simulink model "robot"  (Simulink 9.0)
settings: Solver=FixedStepDiscrete  StartTime=0.0  StopTime=inf  FixedStep=0.022  RelTol=1e-3  EnableMultiTasking=on
values from neighbouring files (symbols this model uses):
  s = zc-d1    [ArticuledManipulator_Ik.m]
undefined symbols (not defined in the file or in its folder): RV
libraries: mblibv1 x37, vrlib x8, simulink x1
settings Model: Creator=Mircea  LastModifiedBy=Rodrigo Chi
settings DataIOCC: LimitDataPoints=on  SignalLoggingSaveFormat=ModelDataLogs
settings OptimizationCC: ExpressionDepthLimit=2147483647
settings DebuggingCC: SolverPrmCheckMsg=warning  FcnCallInpInsideContextMsg=warning  StateNameClashWarn=warning
settings SFSimCC: SimParseCustomCode=off
settings GRTTargetCC: GeneratePreprocessorConditionals=Disable all  CombineOutputUpdateFcns=off  GRTInterface=on
settings ConfigComp: CovSFcnEnable=off
settings SimscapeCC: SimscapeNormalizeSystem=off
settings ConfigurationSet: Description=SimMechanics 2G

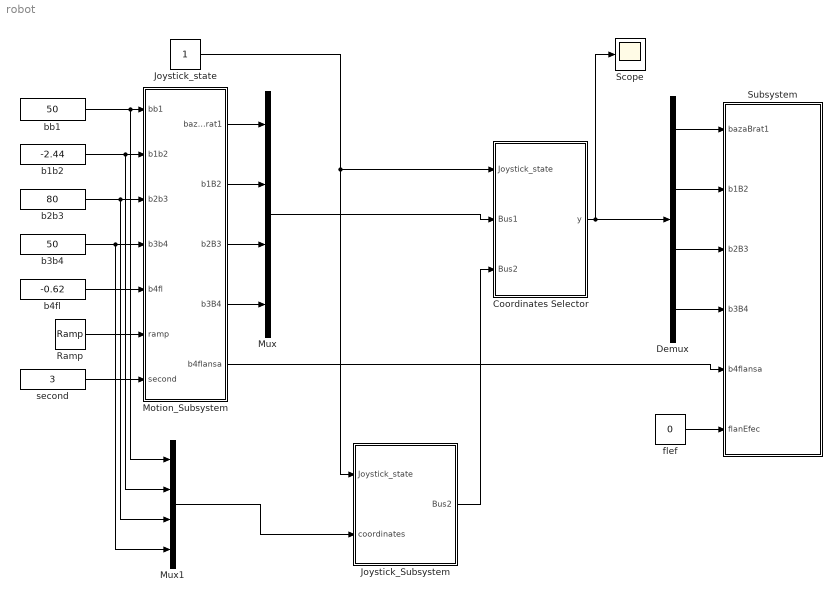
== system robot ==
  "Coordinates Selector " : MATLAB Function  TreatAsAtomicUnit=on
  Demux : Demux
  Joystick_Subsystem : Subsystem
  Joystick_state : Constant
  Motion_Subsystem : Subsystem
  Mux : Mux
  Mux1 : Mux
  Ramp : simulink/Sources/Ramp  slope=25  start=0  X0=0
  Scope : Scope
  Subsystem : Subsystem
  b1b2 : Constant  Value=-2.44
  b2b3 : Constant  Value=80
  b3b4 : Constant  Value=50
  b4fl : Constant  Value=-0.62
  bb1 : Constant  Value=50
  flef : Constant  Value=0
  second : Constant  Value=3
  wires:
  b1b2/1 -> Motion_Subsystem/2(b1b2), Mux1/2
  b2b3/1 -> Motion_Subsystem/3(b2b3), Mux1/3
  b3b4/1 -> Motion_Subsystem/4(b3b4), Mux1/4
  b4fl/1 -> Motion_Subsystem/5(b4fl)
  Ramp/1 -> Motion_Subsystem/6(ramp)
  bb1/1 -> Motion_Subsystem/1(bb1), Mux1/1
  flef/1 -> Subsystem/6(flanEfec)
  second/1 -> Motion_Subsystem/7(second)
  Motion_Subsystem/5(b4flansa) -> Subsystem/5(b4flansa)
  Motion_Subsystem/1(bazaBrat1) -> Mux/1
  Motion_Subsystem/2(b1B2) -> Mux/2
  Motion_Subsystem/3(b2B3) -> Mux/3
  Motion_Subsystem/4(b3B4) -> Mux/4
  Mux/1 -> "Coordinates Selector "/2(Bus1)
  Joystick_state/1 -> "Coordinates Selector "/1(Joystick_state), Joystick_Subsystem/1(Joystick_state)
  "Coordinates Selector "/1(y) -> Demux/1, Scope/1
  Demux/1 -> Subsystem/1(bazaBrat1)
  Demux/2 -> Subsystem/2(b1B2)
  Demux/3 -> Subsystem/3(b2B3)
  Demux/4 -> Subsystem/4(b3B4)
  Mux1/1 -> Joystick_Subsystem/2(coordinates)
  Joystick_Subsystem/1(Bus2) -> "Coordinates Selector "/3(Bus2)

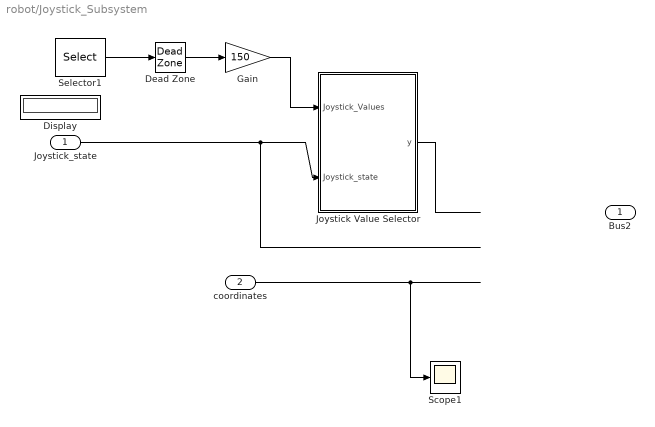
== system robot/Joystick_Subsystem ==
  Joystick_state : Inport
  coordinates : Inport  Port=2
  Dead Zone : DeadZone  SaturateOnIntegerOverflow=on
  Display : Display
  Gain : Gain  Gain=150
  "Joystick Value Selector " : MATLAB Function  TreatAsAtomicUnit=on
  Scope1 : Scope
  Selector1 : Selector  InputPortWidth=8  IndexOptions=Index vector (dialog)  Indices=[1 2 3 4]  OutputSizes=1
  Bus2 : Outport
  wires:
  ? -> Selector1/1
  Selector1/1 -> Dead Zone/1
  Dead Zone/1 -> Gain/1
  coordinates/1 -> Scope1/1
  Joystick_state/1 -> "Joystick Value Selector "/2(Joystick_state)
  Gain/1 -> "Joystick Value Selector "/1(Joystick_Values)
  "Joystick Value Selector "/1(y) -> ?
  ? -> Bus2/1
  ? -> Display/1

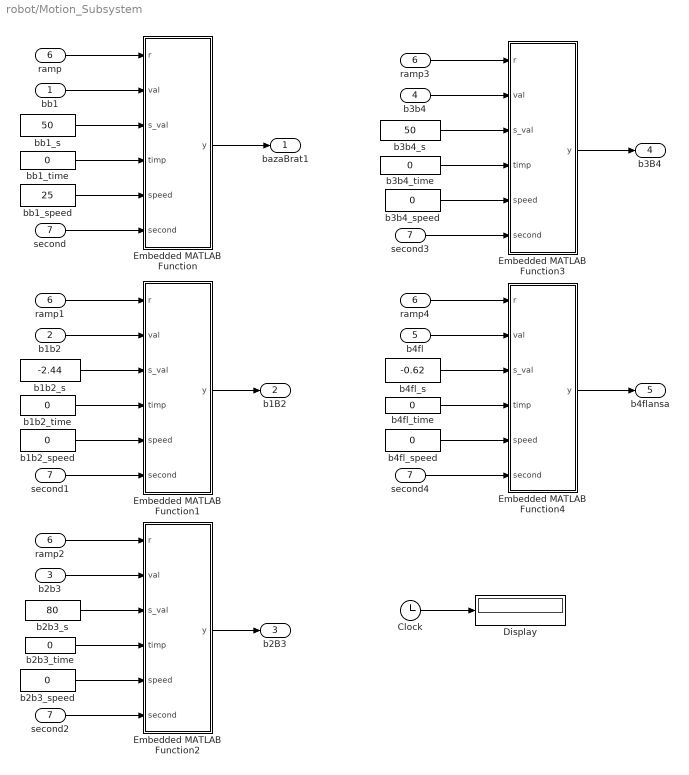
== system robot/Motion_Subsystem ==
  bb1 : Inport
  b1b2 : Inport  Port=2
  b2b3 : Inport  Port=3
  b3b4 : Inport  Port=4
  b4fl : Inport  Port=5
  ramp : Inport  Port=6
  second : Inport  Port=7
  Clock : Clock
  Display : Display
  Embedded MATLAB Function : MATLAB Function  TreatAsAtomicUnit=on
  Embedded MATLAB Function1 : MATLAB Function  TreatAsAtomicUnit=on
  Embedded MATLAB Function2 : MATLAB Function  TreatAsAtomicUnit=on
  Embedded MATLAB Function3 : MATLAB Function  TreatAsAtomicUnit=on
  Embedded MATLAB Function4 : MATLAB Function  TreatAsAtomicUnit=on
  b1b2_s : Constant  Value=-2.44
  b1b2_speed : Constant  Value=0
  b1b2_time : Constant  Value=0
  b2b3_s : Constant  Value=80
  b2b3_speed : Constant  Value=0
  b2b3_time : Constant  Value=0
  b3b4_s : Constant  Value=50
  b3b4_speed : Constant  Value=0
  b3b4_time : Constant  Value=0
  b4fl_s : Constant  Value=-0.62
  b4fl_speed : Constant  Value=0
  b4fl_time : Constant  Value=0
  bb1_s : Constant  Value=50
  bb1_speed : Constant  Value=25
  bb1_time : Constant  Value=0
  ramp{1..4} (4 alike) : InportShadow  Port=6
  second{1..4} (4 alike) : InportShadow  Port=7
  bazaBrat1 : Outport
  b1B2 : Outport  Port=2
  b2B3 : Outport  Port=3
  b3B4 : Outport  Port=4
  b4flansa : Outport  Port=5
  wires:
  ramp/1 -> Embedded MATLAB Function/1(r)
  Clock/1 -> Display/1
  b4fl_time/1 -> Embedded MATLAB Function4/4(timp)
  b4fl_s/1 -> Embedded MATLAB Function4/3(s_val)
  ramp4/1 -> Embedded MATLAB Function4/1(r)
  Embedded MATLAB Function4/1(y) -> b4flansa/1
  b4fl/1 -> Embedded MATLAB Function4/2(val)
  ramp3/1 -> Embedded MATLAB Function3/1(r)
  b3b4_time/1 -> Embedded MATLAB Function3/4(timp)
  b3b4_s/1 -> Embedded MATLAB Function3/3(s_val)
  Embedded MATLAB Function3/1(y) -> b3B4/1
  b3b4/1 -> Embedded MATLAB Function3/2(val)
  b2b3_time/1 -> Embedded MATLAB Function2/4(timp)
  b2b3_s/1 -> Embedded MATLAB Function2/3(s_val)
  ramp2/1 -> Embedded MATLAB Function2/1(r)
  Embedded MATLAB Function2/1(y) -> b2B3/1
  b2b3/1 -> Embedded MATLAB Function2/2(val)
  b1b2_time/1 -> Embedded MATLAB Function1/4(timp)
  b1b2_s/1 -> Embedded MATLAB Function1/3(s_val)
  ramp1/1 -> Embedded MATLAB Function1/1(r)
  Embedded MATLAB Function1/1(y) -> b1B2/1
  b1b2/1 -> Embedded MATLAB Function1/2(val)
  bb1_time/1 -> Embedded MATLAB Function/4(timp)
  bb1_s/1 -> Embedded MATLAB Function/3(s_val)
  Embedded MATLAB Function/1(y) -> bazaBrat1/1
  bb1/1 -> Embedded MATLAB Function/2(val)
  bb1_speed/1 -> Embedded MATLAB Function/5(speed)
  b3b4_speed/1 -> Embedded MATLAB Function3/5(speed)
  b4fl_speed/1 -> Embedded MATLAB Function4/5(speed)
  b2b3_speed/1 -> Embedded MATLAB Function2/5(speed)
  b1b2_speed/1 -> Embedded MATLAB Function1/5(speed)
  second/1 -> Embedded MATLAB Function/6(second)
  second4/1 -> Embedded MATLAB Function4/6(second)
  second3/1 -> Embedded MATLAB Function3/6(second)
  second2/1 -> Embedded MATLAB Function2/6(second)
  second1/1 -> Embedded MATLAB Function1/6(second)

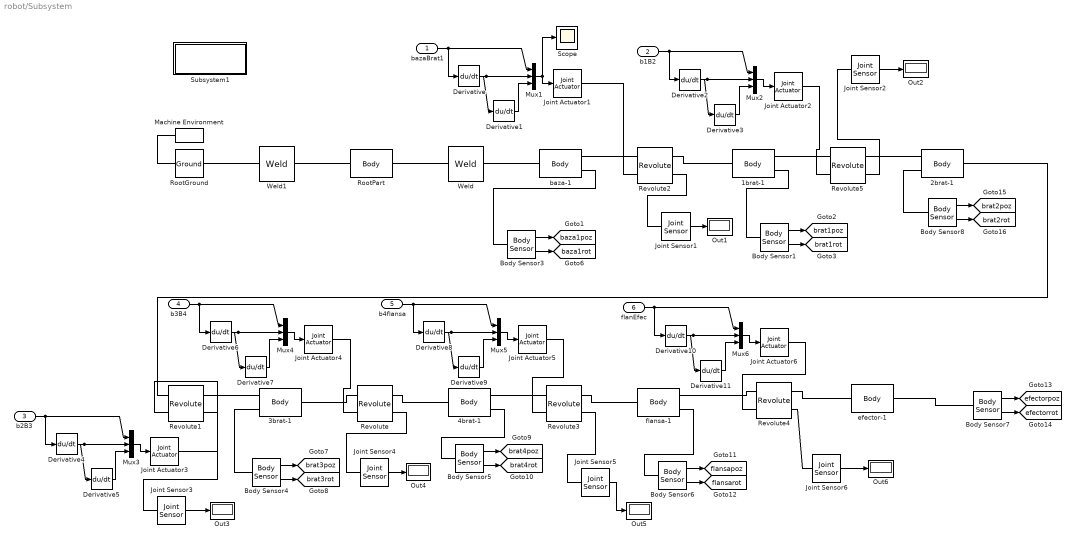
== system robot/Subsystem ==
  bazaBrat1 : Inport
  b1B2 : Inport  Port=2
  b2B3 : Inport  Port=3
  b3B4 : Inport  Port=4
  b4flansa : Inport  Port=5
  flanEfec : Inport  Port=6
  1brat-1 : mblibv1/Bodies/Body  LConnTagsString=CS2  RConnTagsString=CS3|CS4  UpdateFromCAD=on  DialogClass=MechanicalBodyBlock  Mass=2.25015  MassUnits=kg  InertiaUnits=kg*m^2  Inertia=[0.00885227,-5.51348e-008,-0.000219712;-5.51348e-008,0.00930047,6.21532e-009;-0.000219712,6.21532e-009,0.00500541]  Shape=Cylinder  ShapeDims=[1 1]  ShapeUnits=m  ShapeUse=false  Density=1  DensityUnits=kg/m^3  DensityUse=false  GraphicsMode=GFXFILE  GraphicsFileName=robot_nou - 1brat-1.STL  BodyColorSelMode=COLORPALETTE  BodyColor=[0.75294 0.75294 0.75294]  AttachedToCS=CS1  CG=Right$CG$[0.00726331 0.0794388 -8.78869e-008]$WORLD$WORLD$m$[-1 0 0;0 0 1;0 1 0]$3x3 Transform$rad$WORLD$false$none  WorkingFrames=Right$CS1$[0 -0.00299998 0]$WORLD$WORLD$m$[-1 0 0;0 0 1;0 1 0]$3x3 Transform$rad$WORLD$false$none#Left$CS2$[-1.38778e-017 2.5e-008 5.8564e-016]$WORLD$WORLD$m$[1 0 0;0 1 0;0 0 1]$3x3 Transform$rad$WORLD$true$none#Right$CS3$[0 0.1295 -0.0448145]$WORLD$WORLD$m$[1 0 0;0 1 0;0 0 1]$3x3 Transform$rad$WORLD$true$none#Right$CS4$[0 0 0]$WORLD$WORLD$m$[1 0 0;0 1 0;0 0 1]$3x3 Transform$rad$WORLD$true$none  CGPos=[0.00726331 0.0794388 -8.78869e-008]  CGRot=[-1 0 0;0 0 1;0 1 0]  CS0Pos=[]  CS0Rot=[]  CS1Pos=[0 -0.00299998 0]  CS1Rot=[-1 0 0;0 0 1;0 1 0]  CS2Pos=[-1.38778e-017 2.5e-008 5.8564e-016]  CS2Rot=[1 0 0;0 1 0;0 0 1]  CS3Pos=[0 0.1295 -0.0448145]  CS3Rot=[1 0 0;0 1 0;0 0 1]  CS4Pos=[0 0 0]  CS4Rot=[1 0 0;0 1 0;0 0 1]  CS5Pos=[]  CS5Rot=[]  CS6Pos=[]  CS6Rot=[]  CS7Pos=[]  CS7Rot=[]  CS8Pos=[]  CS8Rot=[]  CS9Pos=[]  CS9Rot=[]  CS10Pos=[]  CS10Rot=[]  CS11Pos=[]  CS11Rot=[]  CS12Pos=[]  CS12Rot=[]  CS13Pos=[]  CS13Rot=[]  CS14Pos=[]  CS14Rot=[]  CS15Pos=[]  CS15Rot=[]  CS16Pos=[]  CS16Rot=[]  CS17Pos=[]  CS17Rot=[]  CS18Pos=[]  CS18Rot=[]  CS19Pos=[]  CS19Rot=[]  CS20Pos=[]  CS20Rot=[]
      settings: SourceProductName=Simscape Multibody  SourceProductBaseCode=MS
  2brat-1 : mblibv1/Bodies/Body  LConnTagsString=CS3|CS4  RConnTagsString=CS2  UpdateFromCAD=on  DialogClass=MechanicalBodyBlock  Mass=3.62743  MassUnits=kg  InertiaUnits=kg*m^2  Inertia=[0.0393757,-7.68618e-009,0.000126615;-7.68618e-009,0.0293486,-4.48119e-008;0.000126615,-4.48119e-008,0.0153003]  Shape=Cylinder  ShapeDims=[1 1]  ShapeUnits=m  ShapeUse=false  Density=1  DensityUnits=kg/m^3  DensityUse=false  GraphicsMode=GFXFILE  GraphicsFileName=robot_nou - 2brat-1.STL  BodyColorSelMode=COLORPALETTE  BodyColor=[0.75294 0.75294 0.75294]  AttachedToCS=CS1  CG=Right$CG$[-0.000659844 0.24353 1.10558e-006]$WORLD$WORLD$m$[1 0 0;0 0 1;0 -1 0]$3x3 Transform$rad$WORLD$false$none  WorkingFrames=Right$CS1$[0 0.1295 0]$WORLD$WORLD$m$[1 0 0;0 0 1;0 -1 0]$3x3 Transform$rad$WORLD$false$none#Right$CS2$[0 0.3795 0.0880007]$WORLD$WORLD$m$[1 0 0;0 1 0;0 0 1]$3x3 Transform$rad$WORLD$true$none#Left$CS3$[0 0.1295 -0.0448145]$WORLD$WORLD$m$[1 0 0;0 1 0;0 0 1]$3x3 Transform$rad$WORLD$true$none#Left$CS4$[0 0 0]$WORLD$WORLD$m$[1 0 0;0 1 0;0 0 1]$3x3 Transform$rad$WORLD$true$none  CGPos=[-0.000659844 0.24353 1.10558e-006]  CGRot=[1 0 0;0 0 1;0 -1 0]  CS0Pos=[]  CS0Rot=[]  CS1Pos=[0 0.1295 0]  CS1Rot=[1 0 0;0 0 1;0 -1 0]  CS2Pos=[0 0.3795 0.0880007]  CS2Rot=[1 0 0;0 1 0;0 0 1]  CS3Pos=[0 0.1295 -0.0448145]  CS3Rot=[1 0 0;0 1 0;0 0 1]  CS4Pos=[0 0 0]  CS4Rot=[1 0 0;0 1 0;0 0 1]  CS5Pos=[]  CS5Rot=[]  CS6Pos=[]  CS6Rot=[]  CS7Pos=[]  CS7Rot=[]  CS8Pos=[]  CS8Rot=[]  CS9Pos=[]  CS9Rot=[]  CS10Pos=[]  CS10Rot=[]  CS11Pos=[]  CS11Rot=[]  CS12Pos=[]  CS12Rot=[]  CS13Pos=[]  CS13Rot=[]  CS14Pos=[]  CS14Rot=[]  CS15Pos=[]  CS15Rot=[]  CS16Pos=[]  CS16Rot=[]  CS17Pos=[]  CS17Rot=[]  CS18Pos=[]  CS18Rot=[]  CS19Pos=[]  CS19Rot=[]  CS20Pos=[]  CS20Rot=[]
      settings: SourceProductName=Simscape Multibody  SourceProductBaseCode=MS
  3brat-1 : mblibv1/Bodies/Body  LConnTagsString=CS3|CS4  RConnTagsString=CS2  UpdateFromCAD=on  DialogClass=MechanicalBodyBlock  Mass=1.71089  MassUnits=kg  InertiaUnits=kg*m^2  Inertia=[0.00842552,-6.36697e-007,1.27806e-006;-6.36697e-007,0.00773782,1.23963e-005;1.27806e-006,1.23963e-005,0.00280267]  Shape=Cylinder  ShapeDims=[1 1]  ShapeUnits=m  ShapeUse=false  Density=1  DensityUnits=kg/m^3  DensityUse=false  GraphicsMode=GFXFILE  GraphicsFileName=robot_nou - 3brat-1.STL  BodyColorSelMode=COLORPALETTE  BodyColor=[0.75294 0.75294 0.75294]  AttachedToCS=CS1  CG=Right$CG$[7.52531e-006 0.448063 0.00032452]$WORLD$WORLD$m$[1 0 0;0 0 1;0 -1 0]$3x3 Transform$rad$WORLD$false$none  WorkingFrames=Right$CS1$[0 0.3795 0]$WORLD$WORLD$m$[1 0 0;0 0 1;0 -1 0]$3x3 Transform$rad$WORLD$false$none#Right$CS2$[-0.000180127 0.5395 -0.0224506]$WORLD$WORLD$m$[1 0 0;0 1 0;0 0 1]$3x3 Transform$rad$WORLD$true$none#Left$CS3$[0 0.3795 0.0880007]$WORLD$WORLD$m$[1 0 0;0 1 0;0 0 1]$3x3 Transform$rad$WORLD$true$none#Left$CS4$[0 0 0]$WORLD$WORLD$m$[1 0 0;0 1 0;0 0 1]$3x3 Transform$rad$WORLD$true$none  CGPos=[7.52531e-006 0.448063 0.00032452]  CGRot=[1 0 0;0 0 1;0 -1 0]  CS0Pos=[]  CS0Rot=[]  CS1Pos=[0 0.3795 0]  CS1Rot=[1 0 0;0 0 1;0 -1 0]  CS2Pos=[-0.000180127 0.5395 -0.0224506]  CS2Rot=[1 0 0;0 1 0;0 0 1]  CS3Pos=[0 0.3795 0.0880007]  CS3Rot=[1 0 0;0 1 0;0 0 1]  CS4Pos=[0 0 0]  CS4Rot=[1 0 0;0 1 0;0 0 1]  CS5Pos=[]  CS5Rot=[]  CS6Pos=[]  CS6Rot=[]  CS7Pos=[]  CS7Rot=[]  CS8Pos=[]  CS8Rot=[]  CS9Pos=[]  CS9Rot=[]  CS10Pos=[]  CS10Rot=[]  CS11Pos=[]  CS11Rot=[]  CS12Pos=[]  CS12Rot=[]  CS13Pos=[]  CS13Rot=[]  CS14Pos=[]  CS14Rot=[]  CS15Pos=[]  CS15Rot=[]  CS16Pos=[]  CS16Rot=[]  CS17Pos=[]  CS17Rot=[]  CS18Pos=[]  CS18Rot=[]  CS19Pos=[]  CS19Rot=[]  CS20Pos=[]  CS20Rot=[]
      settings: SourceProductName=Simscape Multibody  SourceProductBaseCode=MS
  4brat-1 : mblibv1/Bodies/Body  LConnTagsString=CS2  RConnTagsString=CS3|CS4  UpdateFromCAD=on  DialogClass=MechanicalBodyBlock  Mass=0.330921  MassUnits=kg  InertiaUnits=kg*m^2  Inertia=[0.000305863,9.08861e-011,-3.82551e-010;9.08861e-011,0.000416962,-1.09526e-009;-3.82551e-010,-1.09526e-009,0.000217954]  Shape=Cylinder  ShapeDims=[1 1]  ShapeUnits=m  ShapeUse=false  Density=1  DensityUnits=kg/m^3  DensityUse=false  GraphicsMode=GFXFILE  GraphicsFileName=robot_nou - 4brat-1.STL  BodyColorSelMode=COLORPALETTE  BodyColor=[0.75294 0.75294 0.75294]  AttachedToCS=CS1  CG=Right$CG$[-0.000180145 0.534322 2.80673e-008]$WORLD$WORLD$m$[1 0 0;0 0 1;0 -1 0]$3x3 Transform$rad$WORLD$false$none  WorkingFrames=Right$CS1$[-0.000180127 0.5395 0]$WORLD$WORLD$m$[1 0 0;0 0 1;0 -1 0]$3x3 Transform$rad$WORLD$false$none#Left$CS2$[-0.000180127 0.5395 -0.0224506]$WORLD$WORLD$m$[1 0 0;0 1 0;0 0 1]$3x3 Transform$rad$WORLD$true$none#Right$CS3$[-0.000180127 0.5855 0]$WORLD$WORLD$m$[1 0 0;0 1 0;0 0 1]$3x3 Transform$rad$WORLD$true$none#Right$CS4$[0 0 0]$WORLD$WORLD$m$[1 0 0;0 1 0;0 0 1]$3x3 Transform$rad$WORLD$true$none  CGPos=[-0.000180145 0.534322 2.80673e-008]  CGRot=[1 0 0;0 0 1;0 -1 0]  CS0Pos=[]  CS0Rot=[]  CS1Pos=[-0.000180127 0.5395 0]  CS1Rot=[1 0 0;0 0 1;0 -1 0]  CS2Pos=[-0.000180127 0.5395 -0.0224506]  CS2Rot=[1 0 0;0 1 0;0 0 1]  CS3Pos=[-0.000180127 0.5855 0]  CS3Rot=[1 0 0;0 1 0;0 0 1]  CS4Pos=[0 0 0]  CS4Rot=[1 0 0;0 1 0;0 0 1]  CS5Pos=[]  CS5Rot=[]  CS6Pos=[]  CS6Rot=[]  CS7Pos=[]  CS7Rot=[]  CS8Pos=[]  CS8Rot=[]  CS9Pos=[]  CS9Rot=[]  CS10Pos=[]  CS10Rot=[]  CS11Pos=[]  CS11Rot=[]  CS12Pos=[]  CS12Rot=[]  CS13Pos=[]  CS13Rot=[]  CS14Pos=[]  CS14Rot=[]  CS15Pos=[]  CS15Rot=[]  CS16Pos=[]  CS16Rot=[]  CS17Pos=[]  CS17Rot=[]  CS18Pos=[]  CS18Rot=[]  CS19Pos=[]  CS19Rot=[]  CS20Pos=[]  CS20Rot=[]
      settings: SourceProductName=Simscape Multibody  SourceProductBaseCode=MS
  Body Sensor{1,3..8} (7 alike) : mblibv1/Sensors &  Actuators/Body Sensor  UpdateFromCAD=off  PhysicalDomain=Mechanical  PortType=blob  Muxed=off  Pose=on  Angle=on  AngleUnits=deg  ArcVelocity=off  ArcVelocityUnits=deg/s  ArcAcceleration=off  ArcAccelerationUnits=deg/s^2  CoordPosition=on  CoordPositionUnits=m  Velocity=off  VelocityUnits=m/s  Acceleration=off  AccelerationUnits=m/s^2  Quaternion=on  QuaternionDT=off  QuaternionDDT=off  QuaternionUnits=off  OutputVector=[1]  ActiveIO=on  Width=12  DialogClass=MechanicalSensorBlock  ReferenceFrame=Absolute (World)
      settings: SourceProductName=Simscape Multibody  SourceProductBaseCode=MS
  Derivative{,1..11} (12 alike) : Derivative
  Joint Actuator{1..6} (6 alike) : mblibv1/Sensors &  Actuators/Joint Actuator  UpdateFromCAD=off  PhysicalDomain=Mechanical  PortType=blob  ActuationStyle=Motion  AngleUnits=deg  ArcVelocityUnits=deg/s  ArcAccelerationUnits=deg/s^2  CoordPositionUnits=m  VelocityUnits=m/s  AccelerationUnits=m/s^2  ForceUnits=N  TorqueUnits=N*m  ActiveIO=on  Width=3  DialogClass=MechanicalActuatorBlock  Primitive=R1  ReferenceFrame=Absolute (World)
      settings: SourceProductName=Simscape Multibody  SourceProductBaseCode=MS
  Joint Sensor{1..6} (6 alike) : mblibv1/Sensors &  Actuators/Joint Sensor  UpdateFromCAD=off  PhysicalDomain=Mechanical  PortType=blob  Muxed=on  Pose=off  Angle=on  AngleUnits=deg  ArcVelocity=off  ArcVelocityUnits=deg/s  ArcAcceleration=off  ArcAccelerationUnits=deg/s^2  CoordPosition=on  CoordPositionUnits=m  Velocity=off  VelocityUnits=m/s  Acceleration=off  AccelerationUnits=m/s^2  Quaternion=on  QuaternionDT=off  QuaternionDDT=off  QuaternionUnits=off  OutputVector=[1]  ActiveIO=on  Width=1  DialogClass=MechanicalSensorBlock  Primitive=R1  Force=off  ForceUnits=N  Torque=off  TorqueUnits=N-m  ReferenceFrame=Absolute (World)  ReactionSensedSide=Base  ReactionReferenceFrame=Absolute (World)  ReactionForce=off  ReactionForceUnits=N  ReactionMoment=off  ReactionMomentUnits=N-m
      settings: SourceProductName=Simscape Multibody  SourceProductBaseCode=MS
  Machine Environment : mblibv1/Bodies/Machine Environment  PortType=env  PhysicalDomain=Mechanical  DialogTemplateClass=MECH.MachineEnvironment  SyncWhenCopied=off  Gravity=[0 -9.81 0]  GravityUnits=m/s^2  GravityAsSignal=off  Dimensionality=Auto-detect  AnalysisType=Forward dynamics  LinearAssemblyTolerance=1e-3  LinearAssemblyToleranceUnits=m  AngularAssemblyTolerance=1e-3  AngularAssemblyToleranceUnits=rad  ConstraintSolverType=Stabilizing  ConstraintRelTolerance=1e-4  ConstraintAbsTolerance=1e-4  UseRobustSingularityHandling=off  RedundancyAnalysisToleranceType=Automatically select tolerance  RedundancyAnalysisTolerance=1e-14  StatePerturbationType=Fixed  PerturbationSize=1e-5  VisualizeMachine=on  BodyVisualizationType=Use model default body geometries  BodyColorSelMode=Use model default  DefaultBodyColor=[1 0 0]
      settings: SourceProductName=Simscape Multibody  SourceProductBaseCode=MS
  Mux{1..6} (6 alike) : Mux  Inputs=3
  Out{1..6} (6 alike) : Display
  Revolute : mblibv1/Joints/Revolute  LConnTagsString=__newl0|SA1  RConnTagsString=__newr0|SA1  UpdateFromCAD=on  NumSAPorts=2  CutJoint=off  MarkAsCut=off  Primitives=prismatic  PrimitiveProps=R1$World$[0,0,-1]$revolute  DialogClass=JointBlock  R1Axis=[0,0,-1]
      settings: SourceProductName=Simscape Multibody  SourceProductBaseCode=MS
  Revolute1 : mblibv1/Joints/Revolute  LConnTagsString=__newl0|SA1  RConnTagsString=__newr0|SA1  UpdateFromCAD=on  NumSAPorts=2  CutJoint=off  MarkAsCut=off  Primitives=prismatic  PrimitiveProps=R1$World$[0,0,-1]$revolute  DialogClass=JointBlock  R1Axis=[0,0,-1]
      settings: SourceProductName=Simscape Multibody  SourceProductBaseCode=MS
  Revolute2 : mblibv1/Joints/Revolute  LConnTagsString=__newl0|SA1  RConnTagsString=__newr0|SA1  UpdateFromCAD=on  NumSAPorts=2  CutJoint=off  MarkAsCut=off  Primitives=prismatic  PrimitiveProps=R1$World$[0,1,0]$revolute  DialogClass=JointBlock  R1Axis=[0,1,0]
      settings: SourceProductName=Simscape Multibody  SourceProductBaseCode=MS
  Revolute3 : mblibv1/Joints/Revolute  LConnTagsString=__newl0|SA1  RConnTagsString=__newr0|SA1  UpdateFromCAD=on  NumSAPorts=2  CutJoint=off  MarkAsCut=off  Primitives=prismatic  PrimitiveProps=R1$World$[0,1,0]$revolute  DialogClass=JointBlock  R1Axis=[0,1,0]
      settings: SourceProductName=Simscape Multibody  SourceProductBaseCode=MS
  Revolute4 : mblibv1/Joints/Revolute  LConnTagsString=__newl0|SA1  RConnTagsString=__newr0|SA1  UpdateFromCAD=on  NumSAPorts=2  CutJoint=off  MarkAsCut=off  Primitives=prismatic  PrimitiveProps=R1$World$[0,1,0]$revolute  DialogClass=JointBlock  R1Axis=[0,1,0]
      settings: SourceProductName=Simscape Multibody  SourceProductBaseCode=MS
  Revolute5 : mblibv1/Joints/Revolute  LConnTagsString=__newl0|SA1  RConnTagsString=__newr0|SA1  UpdateFromCAD=on  NumSAPorts=2  CutJoint=off  MarkAsCut=off  Primitives=prismatic  PrimitiveProps=R1$World$[0,0,1]$revolute  DialogClass=JointBlock  R1Axis=[0,0,1]
      settings: SourceProductName=Simscape Multibody  SourceProductBaseCode=MS
  RootGround : mblibv1/Bodies/Ground  UpdateFromCAD=on  LeftPortType=env  RightPortType=workingframe  PhysicalDomain=Mechanical  DialogClass=GroundBlock  CoordPosition=[0.0162361,0.125438,4.43298e-005]  CoordPositionUnits=m  StateVectorMgrId=0  MachineId=[1 0]  ShowEnvPort=on  ParameterChecksum=[818060553, 459790774, 296040721, 266465666]  TopologyChecksum=[932348665, 1302683671, 228289531, 2549500922]
      settings: SourceProductName=Simscape Multibody  SourceProductBaseCode=MS
  RootPart : mblibv1/Bodies/Body  LConnTagsString=CS3  RConnTagsString=CS2  UpdateFromCAD=on  DialogClass=MechanicalBodyBlock  Mass=0  MassUnits=kg  InertiaUnits=kg*m^2  Inertia=[0,0,0;0,0,0;0,0,0]  Shape=Cylinder  ShapeDims=[1 1]  ShapeUnits=m  ShapeUse=false  Density=1  DensityUnits=kg/m^3  DensityUse=false  GraphicsMode=MACHINE_DEFAULT  BodyColorSelMode=MACHINE_DEFAULT  BodyColor=[1;0;0]  AttachedToCS=CS1  CG=Right$CG$[0.0162361 0.125438 4.43298e-005]$WORLD$WORLD$m$[1 0 0;0 1 0;0 0 1]$3x3 Transform$rad$WORLD$false$none  WorkingFrames=Right$CS1$[0 0 0]$WORLD$WORLD$m$[1 0 0;0 1 0;0 0 1]$3x3 Transform$rad$WORLD$false$none#Right$CS2$[0.0387863 -0.0914613 7.26852e-006]$WORLD$WORLD$m$[1 0 0;0 1 0;0 0 1]$3x3 Transform$rad$WORLD$true$none#Left$CS3$[0.0162361 0.125438 4.43298e-005]$WORLD$WORLD$m$[1 0 0;0 1 0;0 0 1]$3x3 Transform$rad$WORLD$true$none  CGPos=[0.0162361 0.125438 4.43298e-005]  CGRot=[1 0 0;0 1 0;0 0 1]  CS0Pos=[]  CS0Rot=[]  CS1Pos=[0 0 0]  CS1Rot=[1 0 0;0 1 0;0 0 1]  CS2Pos=[0.0387863 -0.0914613 7.26852e-006]  CS2Rot=[1 0 0;0 1 0;0 0 1]  CS3Pos=[0.0162361 0.125438 4.43298e-005]  CS3Rot=[1 0 0;0 1 0;0 0 1]  CS4Pos=[]  CS4Rot=[]  CS5Pos=[]  CS5Rot=[]  CS6Pos=[]  CS6Rot=[]  CS7Pos=[]  CS7Rot=[]  CS8Pos=[]  CS8Rot=[]  CS9Pos=[]  CS9Rot=[]  CS10Pos=[]  CS10Rot=[]  CS11Pos=[]  CS11Rot=[]  CS12Pos=[]  CS12Rot=[]  CS13Pos=[]  CS13Rot=[]  CS14Pos=[]  CS14Rot=[]  CS15Pos=[]  CS15Rot=[]  CS16Pos=[]  CS16Rot=[]  CS17Pos=[]  CS17Rot=[]  CS18Pos=[]  CS18Rot=[]  CS19Pos=[]  CS19Rot=[]  CS20Pos=[]  CS20Rot=[]
      settings: SourceProductName=Simscape Multibody  SourceProductBaseCode=MS
  Scope : Scope
  Subsystem1 : Subsystem
  Weld : mblibv1/Joints/Weld  LConnTagsString=__newl0  RConnTagsString=__newr0  UpdateFromCAD=on  NumSAPorts=0  CutJoint=off  MarkAsCut=off  Primitives=weld  PrimitiveProps=W$WORLD$[0.57735,0.57735,0.57735]$weld  DialogClass=JointBlock  WAxis=[0.57735,0.57735,0.57735]
      settings: SourceProductName=Simscape Multibody  SourceProductBaseCode=MS
  Weld1 : mblibv1/Joints/Weld  LConnTagsString=__newl0  RConnTagsString=__newr0  UpdateFromCAD=on  NumSAPorts=0  CutJoint=off  MarkAsCut=off  Primitives=weld  PrimitiveProps=W$WORLD$[0.57735,0.57735,0.57735]$weld  DialogClass=JointBlock  WAxis=[0.57735,0.57735,0.57735]
      settings: SourceProductName=Simscape Multibody  SourceProductBaseCode=MS
  baza-1 : mblibv1/Bodies/Body  LConnTagsString=CS2  RConnTagsString=CS3|CS4  UpdateFromCAD=on  DialogClass=MechanicalBodyBlock  Mass=5.28442  MassUnits=kg  InertiaUnits=kg*m^2  Inertia=[0.0219514,4.64467e-006,-0.00187329;4.64467e-006,0.0327268,7.62797e-007;-0.00187329,7.62797e-007,0.0305246]  Shape=Cylinder  ShapeDims=[1 1]  ShapeUnits=m  ShapeUse=false  Density=1  DensityUnits=kg/m^3  DensityUse=false  GraphicsMode=GFXFILE  GraphicsFileName=robot_nou - baza-1.STL  BodyColorSelMode=COLORPALETTE  BodyColor=[0.75294 0.75294 0.75294]  AttachedToCS=CS1  CG=Right$CG$[0.0387863 -0.0914613 7.26852e-006]$WORLD$WORLD$m$[-1 0 0;0 0 1;0 1 0]$3x3 Transform$rad$WORLD$false$none  WorkingFrames=Right$CS1$[0 -0.168 0]$WORLD$WORLD$m$[-1 0 0;0 0 1;0 1 0]$3x3 Transform$rad$WORLD$false$none#Left$CS2$[0.0387863 -0.0914613 7.26852e-006]$WORLD$WORLD$m$[1 0 0;0 1 0;0 0 1]$3x3 Transform$rad$WORLD$true$none#Right$CS3$[-1.38778e-017 2.5e-008 5.8564e-016]$WORLD$WORLD$m$[1 0 0;0 1 0;0 0 1]$3x3 Transform$rad$WORLD$true$none#Right$CS4$[0 0 0]$WORLD$WORLD$m$[1 0 0;0 1 0;0 0 1]$3x3 Transform$rad$WORLD$true$none  CGPos=[0.0387863 -0.0914613 7.26852e-006]  CGRot=[-1 0 0;0 0 1;0 1 0]  CS0Pos=[]  CS0Rot=[]  CS1Pos=[0 -0.168 0]  CS1Rot=[-1 0 0;0 0 1;0 1 0]  CS2Pos=[0.0387863 -0.0914613 7.26852e-006]  CS2Rot=[1 0 0;0 1 0;0 0 1]  CS3Pos=[-1.38778e-017 2.5e-008 5.8564e-016]  CS3Rot=[1 0 0;0 1 0;0 0 1]  CS4Pos=[0 0 0]  CS4Rot=[1 0 0;0 1 0;0 0 1]  CS5Pos=[]  CS5Rot=[]  CS6Pos=[]  CS6Rot=[]  CS7Pos=[]  CS7Rot=[]  CS8Pos=[]  CS8Rot=[]  CS9Pos=[]  CS9Rot=[]  CS10Pos=[]  CS10Rot=[]  CS11Pos=[]  CS11Rot=[]  CS12Pos=[]  CS12Rot=[]  CS13Pos=[]  CS13Rot=[]  CS14Pos=[]  CS14Rot=[]  CS15Pos=[]  CS15Rot=[]  CS16Pos=[]  CS16Rot=[]  CS17Pos=[]  CS17Rot=[]  CS18Pos=[]  CS18Rot=[]  CS19Pos=[]  CS19Rot=[]  CS20Pos=[]  CS20Rot=[]
      settings: SourceProductName=Simscape Multibody  SourceProductBaseCode=MS
  efector-1 : mblibv1/Bodies/Body  LConnTagsString=CS2  RConnTagsString=CS3  UpdateFromCAD=on  DialogClass=MechanicalBodyBlock  Mass=0.170431  MassUnits=kg  InertiaUnits=kg*m^2  Inertia=[0.000106215,-1.25677e-006,2.43146e-015;-1.25677e-006,0.00010751,1.48259e-015;2.43146e-015,1.48259e-015,0.000156336]  Shape=Cylinder  ShapeDims=[1 1]  ShapeUnits=m  ShapeUse=false  Density=1  DensityUnits=kg/m^3  DensityUse=false  GraphicsMode=GFXFILE  GraphicsFileName=robot_nou - efector-1.STL  BodyColorSelMode=COLORPALETTE  BodyColor=[1 0.50196 0.50196]  AttachedToCS=CS1  CG=Right$CG$[-0.000180127 0.62715 0]$WORLD$WORLD$m$[1 0 0;0 0 1;0 -1 0]$3x3 Transform$rad$WORLD$false$none  WorkingFrames=Right$CS1$[-0.000180127 0.6048 0]$WORLD$WORLD$m$[1 0 0;0 0 1;0 -1 0]$3x3 Transform$rad$WORLD$false$none#Left$CS2$[-0.000180127 0.6048 0]$WORLD$WORLD$m$[1 0 0;0 1 0;0 0 1]$3x3 Transform$rad$WORLD$true$none#Right$CS3$[0 0 0]$WORLD$WORLD$m$[1 0 0;0 1 0;0 0 1]$3x3 Transform$rad$WORLD$true$none  CGPos=[-0.000180127 0.62715 0]  CGRot=[1 0 0;0 0 1;0 -1 0]  CS0Pos=[]  CS0Rot=[]  CS1Pos=[-0.000180127 0.6048 0]  CS1Rot=[1 0 0;0 0 1;0 -1 0]  CS2Pos=[-0.000180127 0.6048 0]  CS2Rot=[1 0 0;0 1 0;0 0 1]  CS3Pos=[0 0 0]  CS3Rot=[1 0 0;0 1 0;0 0 1]  CS4Pos=[]  CS4Rot=[]  CS5Pos=[]  CS5Rot=[]  CS6Pos=[]  CS6Rot=[]  CS7Pos=[]  CS7Rot=[]  CS8Pos=[]  CS8Rot=[]  CS9Pos=[]  CS9Rot=[]  CS10Pos=[]  CS10Rot=[]  CS11Pos=[]  CS11Rot=[]  CS12Pos=[]  CS12Rot=[]  CS13Pos=[]  CS13Rot=[]  CS14Pos=[]  CS14Rot=[]  CS15Pos=[]  CS15Rot=[]  CS16Pos=[]  CS16Rot=[]  CS17Pos=[]  CS17Rot=[]  CS18Pos=[]  CS18Rot=[]  CS19Pos=[]  CS19Rot=[]  CS20Pos=[]  CS20Rot=[]
      settings: SourceProductName=Simscape Multibody  SourceProductBaseCode=MS
  flansa-1 : mblibv1/Bodies/Body  LConnTagsString=CS2  RConnTagsString=CS3|CS4  UpdateFromCAD=on  DialogClass=MechanicalBodyBlock  Mass=0.103138  MassUnits=kg  InertiaUnits=kg*m^2  Inertia=[4.34781e-005,0,-2.81871e-008;0,4.34391e-005,0;-2.81871e-008,0,7.89834e-005]  Shape=Cylinder  ShapeDims=[1 1]  ShapeUnits=m  ShapeUse=false  Density=1  DensityUnits=kg/m^3  DensityUse=false  GraphicsMode=GFXFILE  GraphicsFileName=robot_nou - flansa-1.STL  BodyColorSelMode=COLORPALETTE  BodyColor=[0.75294 0.75294 0.75294]  AttachedToCS=CS1  CG=Right$CG$[-0.00015614 0.595907 0]$WORLD$WORLD$m$[1 0 0;0 0 1;0 -1 0]$3x3 Transform$rad$WORLD$false$none  WorkingFrames=Right$CS1$[-0.000180127 0.6113 0]$WORLD$WORLD$m$[1 0 0;0 0 1;0 -1 0]$3x3 Transform$rad$WORLD$false$none#Left$CS2$[-0.000180127 0.5855 0]$WORLD$WORLD$m$[1 0 0;0 1 0;0 0 1]$3x3 Transform$rad$WORLD$true$none#Right$CS3$[-0.000180127 0.6048 0]$WORLD$WORLD$m$[1 0 0;0 1 0;0 0 1]$3x3 Transform$rad$WORLD$true$none#Right$CS4$[0 0 0]$WORLD$WORLD$m$[1 0 0;0 1 0;0 0 1]$3x3 Transform$rad$WORLD$true$none  CGPos=[-0.00015614 0.595907 0]  CGRot=[1 0 0;0 0 1;0 -1 0]  CS0Pos=[]  CS0Rot=[]  CS1Pos=[-0.000180127 0.6113 0]  CS1Rot=[1 0 0;0 0 1;0 -1 0]  CS2Pos=[-0.000180127 0.5855 0]  CS2Rot=[1 0 0;0 1 0;0 0 1]  CS3Pos=[-0.000180127 0.6048 0]  CS3Rot=[1 0 0;0 1 0;0 0 1]  CS4Pos=[0 0 0]  CS4Rot=[1 0 0;0 1 0;0 0 1]  CS5Pos=[]  CS5Rot=[]  CS6Pos=[]  CS6Rot=[]  CS7Pos=[]  CS7Rot=[]  CS8Pos=[]  CS8Rot=[]  CS9Pos=[]  CS9Rot=[]  CS10Pos=[]  CS10Rot=[]  CS11Pos=[]  CS11Rot=[]  CS12Pos=[]  CS12Rot=[]  CS13Pos=[]  CS13Rot=[]  CS14Pos=[]  CS14Rot=[]  CS15Pos=[]  CS15Rot=[]  CS16Pos=[]  CS16Rot=[]  CS17Pos=[]  CS17Rot=[]  CS18Pos=[]  CS18Rot=[]  CS19Pos=[]  CS19Rot=[]  CS20Pos=[]  CS20Rot=[]
      settings: SourceProductName=Simscape Multibody  SourceProductBaseCode=MS
  tag scope: baza1poz=global, baza1rot=global, brat1poz=global, brat1rot=global, brat2poz=global, brat2rot=global, brat3poz=global, brat3rot=global, brat4poz=global, brat4rot=global, efectorpoz=global, efectorrot=global, flansapoz=global, flansarot=global
  wires:
  Body Sensor3/2 -> [baza1rot]
  Body Sensor3/1 -> [baza1poz]
  Body Sensor1/2 -> [brat1rot]
  Body Sensor1/1 -> [brat1poz]
  Body Sensor4/2 -> [brat3rot]
  Body Sensor4/1 -> [brat3poz]
  Body Sensor5/2 -> [brat4rot]
  Body Sensor5/1 -> [brat4poz]
  Body Sensor6/2 -> [flansarot]
  Body Sensor6/1 -> [flansapoz]
  Body Sensor7/2 -> [efectorrot]
  Body Sensor7/1 -> [efectorpoz]
  Mux1/1 -> Joint Actuator1/1, Scope/1
  bazaBrat1/1 -> Derivative/1, Mux1/1
  Derivative/1 -> Derivative1/1, Mux1/2
  Derivative1/1 -> Mux1/3
  Joint Sensor1/1 -> Out1/1
  Mux2/1 -> Joint Actuator2/1
  b1B2/1 -> Derivative2/1, Mux2/1
  Derivative2/1 -> Derivative3/1, Mux2/2
  Derivative3/1 -> Mux2/3
  Joint Sensor2/1 -> Out2/1
  Mux3/1 -> Joint Actuator3/1
  b2B3/1 -> Derivative4/1, Mux3/1
  Derivative4/1 -> Derivative5/1, Mux3/2
  Derivative5/1 -> Mux3/3
  Joint Sensor3/1 -> Out3/1
  Mux4/1 -> Joint Actuator4/1
  b3B4/1 -> Derivative6/1, Mux4/1
  Derivative6/1 -> Derivative7/1, Mux4/2
  Derivative7/1 -> Mux4/3
  Joint Sensor4/1 -> Out4/1
  Mux5/1 -> Joint Actuator5/1
  b4flansa/1 -> Mux5/1, Derivative8/1
  Derivative8/1 -> Mux5/2, Derivative9/1
  Derivative9/1 -> Mux5/3
  Joint Sensor5/1 -> Out5/1
  Joint Sensor6/1 -> Out6/1
  Mux6/1 -> Joint Actuator6/1
  flanEfec/1 -> Derivative10/1, Mux6/1
  Derivative10/1 -> Derivative11/1, Mux6/2
  Derivative11/1 -> Mux6/3
  Body Sensor8/2 -> [brat2rot]
  Body Sensor8/1 -> [brat2poz]
  connections:
  baza-1/RConn1 -- Revolute2/LConn1
  Revolute/RConn1 -- 4brat-1/LConn1
  1brat-1/RConn1 -- Revolute5/LConn1
  Revolute1/RConn1 -- 3brat-1/LConn1
  Revolute3/RConn1 -- flansa-1/LConn1
  RootGround/RConn1 -- Weld1/LConn1
  Revolute4/RConn1 -- efector-1/LConn1
  4brat-1/RConn1 -- Revolute3/LConn1
  Weld1/RConn1 -- RootPart/LConn1
  flansa-1/RConn1 -- Revolute4/LConn1
  Revolute5/RConn1 -- 2brat-1/LConn1
  Weld/RConn1 -- baza-1/LConn1
  RootPart/RConn1 -- Weld/LConn1
  RootGround/LConn1 -- Machine Environment/RConn1
  2brat-1/RConn1 -- Revolute1/LConn1
  Revolute2/RConn1 -- 1brat-1/LConn1
  3brat-1/RConn1 -- Revolute/LConn1
  Joint Sensor6/LConn1 -- Revolute4/RConn2
  Joint Actuator6/RConn1 -- Revolute4/LConn2
  Body Sensor7/LConn1 -- efector-1/RConn1
  flansa-1/RConn2 -- Body Sensor6/LConn1
  Revolute3/RConn2 -- Joint Sensor5/LConn1
  Joint Actuator5/RConn1 -- Revolute3/LConn2
  4brat-1/RConn2 -- Body Sensor5/LConn1
  Joint Sensor4/LConn1 -- Revolute/RConn2
  Joint Actuator4/RConn1 -- Revolute/LConn2
  3brat-1/LConn2 -- Body Sensor4/LConn1
  Revolute1/LConn2 -- Joint Actuator3/RConn1
  Joint Sensor3/LConn1 -- Revolute1/RConn2
  Body Sensor8/LConn1 -- 2brat-1/LConn2
  Joint Sensor2/LConn1 -- Revolute5/RConn2
  Joint Actuator2/RConn1 -- Revolute5/LConn2
  Body Sensor1/LConn1 -- 1brat-1/RConn2
  Joint Actuator1/RConn1 -- Revolute2/LConn2
  Joint Sensor1/LConn1 -- Revolute2/RConn2
  Body Sensor3/LConn1 -- baza-1/RConn2

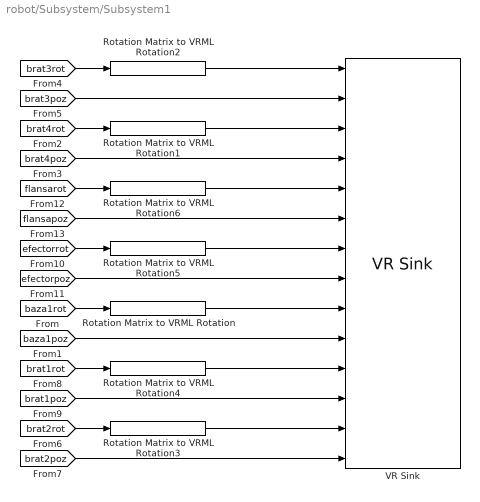
== system robot/Subsystem/Subsystem1 ==
  Rotation Matrix to VRML Rotation{,1..6} (7 alike) : vrlib/Utilities/Rotation Matrix to VRML Rotation  maxzero=1e-12
      settings: SourceProductName=Simulink 3D Animation  SourceProductBaseCode=VR
  VR Sink : vrlib/VR Sink  InstantiateOnLoad=on  SampleTime=0.022  ViewEnable=on  RemoteChange=off  RemoteView=on  FieldsWritten=b3.rotation.4.1.double#b3.translation.3.1.double#b4.rotation.4.1.double#b4.translation.3.1.double#f.rotation.4.1.double#f.translation.3.1.double#e.rotation.4.1.double#e.translation.3.1.double#bb.rotation.4.1.double#bb.translation.3.1.double#b1.rotation.4.1.double#b1.translation.3.1.double#b2.rotation.4.1.double#b2.translation.3.1.double  WorldFileName=robot_nou.wrl  WorldDescription=RV-2AJ  AutoView=off  VideoDimensions=[]  AllowVariableSize=off
      settings: SourceProductBaseCode=VR
  wires:
  [baza1rot] -> Rotation Matrix to VRML Rotation/1
  [brat4rot] -> Rotation Matrix to VRML Rotation1/1
  [brat3rot] -> Rotation Matrix to VRML Rotation2/1
  [brat2rot] -> Rotation Matrix to VRML Rotation3/1
  [brat1rot] -> Rotation Matrix to VRML Rotation4/1
  [efectorrot] -> Rotation Matrix to VRML Rotation5/1
  [flansarot] -> Rotation Matrix to VRML Rotation6/1
  Rotation Matrix to VRML Rotation2/1 -> VR Sink/1
  [brat3poz] -> VR Sink/2
  Rotation Matrix to VRML Rotation1/1 -> VR Sink/3
  [brat4poz] -> VR Sink/4
  Rotation Matrix to VRML Rotation6/1 -> VR Sink/5
  [flansapoz] -> VR Sink/6
  Rotation Matrix to VRML Rotation5/1 -> VR Sink/7
  [efectorpoz] -> VR Sink/8
  Rotation Matrix to VRML Rotation/1 -> VR Sink/9
  [baza1poz] -> VR Sink/10
  Rotation Matrix to VRML Rotation4/1 -> VR Sink/11
  [brat1poz] -> VR Sink/12
  Rotation Matrix to VRML Rotation3/1 -> VR Sink/13
  [brat2poz] -> VR Sink/14

== matlab function Motion_Subsystem/Embedded MATLAB Function ==
  data: r input double; y output double; val input double; s_val input double; timp input double; speed input double; second input double
function y = fcn(r,val,s_val,timp,speed,second)
%#eml
eml.extrinsic('set_param');
eml.extrinsic('num2str');
if val-s_val~=0
    if r<timp+second
      if val-s_val>=0
        yf=s_val+(r-timp)*speed;
      else
        yf=s_val-(r-timp)*speed;
      end
    else
       yf=val;
       set_param('robot/Motion_Subsystem/bb1_s','Value',num2str(val));
    end
else
    yf=val;
    set_param('robot/Motion_Subsystem/bb1_s','Value',num2str(val))
end;
y=yf;

== matlab function Coordinates Selector  ==
  data: Joystick_state input double; y output double; Bus1 input double; Bus2 input double
function y = fcn(Joystick_state,Bus1,Bus2)
%#eml
if Joystick_state==1
    y1=Bus1;
else
    y1=Bus1;
end;
y = y1;

== matlab function Motion_Subsystem/Embedded MATLAB Function1 ==
  data: r input double; y output double; val input double; s_val input double; timp input double; speed input double; second input double
function y = fcn(r,val,s_val,timp,speed,second)
%#eml
eml.extrinsic('set_param');
eml.extrinsic('num2str');
if val-s_val~=0
    if r<timp+second
      if val-s_val>=0
        yf=s_val+(r-timp)*speed;
      else
        yf=s_val-(r-timp)*speed;
      end
    else
       yf=val;
       set_param('robot/Motion_Subsystem/b1b2_s','Value',num2str(val));
    end
else
    yf=val;
    set_param('robot/Motion_Subsystem/b1b2_s','Value',num2str(val))
end;
y=yf;

== matlab function Motion_Subsystem/Embedded MATLAB Function2 ==
  data: r input double; y output double; val input double; s_val input double; timp input double; speed input double; second input double
function y = fcn(r,val,s_val,timp,speed,second)
%#eml
eml.extrinsic('set_param');
eml.extrinsic('num2str');
if val-s_val~=0
    if r<timp+second
      if val-s_val>=0
        yf=s_val+(r-timp)*speed;
      else
        yf=s_val-(r-timp)*speed;
      end
    else
       yf=val;
       set_param('robot/Motion_Subsystem/b2b3_s','Value',num2str(val));
    end
else
    yf=val;
    set_param('robot/Motion_Subsystem/b2b3_s','Value',num2str(val))
end;
y=yf;

== matlab function Motion_Subsystem/Embedded MATLAB Function3 ==
  data: r input double; y output double; val input double; s_val input double; timp input double; speed input double; second input double
function y = fcn(r,val,s_val,timp,speed,second)
%#eml
eml.extrinsic('set_param');
eml.extrinsic('num2str');
if val-s_val~=0
    if r<timp+second
      if val-s_val>=0
        yf=s_val+(r-timp)*speed;
      else
        yf=s_val-(r-timp)*speed;
      end
    else
       yf=val;
       set_param('robot/Motion_Subsystem/b3b4_s','Value',num2str(val));
    end
else
    yf=val;
    set_param('robot/Motion_Subsystem/b3b4_s','Value',num2str(val))
end;
y=yf;

== matlab function Motion_Subsystem/Embedded MATLAB Function4 ==
  data: r input double; y output double; val input double; s_val input double; timp input double; speed input double; second input double
function y = fcn(r,val,s_val,timp,speed,second)
%#eml
eml.extrinsic('set_param');
eml.extrinsic('num2str');
if val-s_val~=0
    if r<timp+second
      if val-s_val>=0
        yf=s_val+(r-timp)*speed;
      else
        yf=s_val-(r-timp)*speed;
      end
    else
       yf=val;
       set_param('robot/Motion_Subsystem/b4fl_s','Value',num2str(val));
    end
else
    yf=val;
    set_param('robot/Motion_Subsystem/b4fl_s','Value',num2str(val))
end;
y=yf;

== matlab function Joystick_Subsystem/Joystick Value Selector  ==
  data: Joystick_Values input double; Joystick_state input double; y output double
function y = fcn(Joystick_Values,Joystick_state)
%#eml
if Joystick_state==1
    y1=Joystick_Values;
else
    y1=[0;0;0;0];
end;
y = y1;
